simulink model "SWC_TPMS_APS_type"  (R2021b)
settings: Solver=FixedStepDiscrete  StartTime=0.0  StopTime=10.0  FixedStep=0.001  RelTol=1e-3
undefined symbols (not defined in the file or in its folder): f32_ApsOutVehSpdSig, R_HALIN_TPMS_APS_CSOP_PAS_Handler, R_HALIN_TPMS_APS_CSOP_TPMS_Handler, R_HALOUT_TPMS_APS_CSOP_ApsOutput, u8_ApsOutGearPosnSig, u8_ApsOutSendChrgPlugSta, u8_ApsOutSetFrSensorOnCmd, u8_ApsOutSetFrSensorSwTOCmd, u8_ApsOutSetVehSpdTOCmd
(part 1 of 2)
settings Model: DataDictionary=APPTypes.sldd  Creator=FVT23010  LastModifiedBy=FVT23010
settings DataIOCC: SaveFormat=StructureWithTime
settings OptimizationCC: DefaultParameterBehavior=Inlined  EnhancedBackFolding=on  PassReuseOutputArgsAs=Individual arguments  ZeroExternalMemoryAtStartup=off  ZeroInternalMemoryAtStartup=off  OptimizeBlockOrder=speed  DifferentSizesBufferReuse=on  OptimizationCustomize=off  EfficientTunableParamExpr=on
settings DebuggingCC: ParameterTunabilityLossMsg=error
settings HardwareCC: ProdBitPerPointer=32  ProdBitPerSizeT=32  ProdBitPerPtrDiffT=32  ProdLargestAtomicInteger=Long  ProdLargestAtomicFloat=Double  ProdWordSize=32  ProdLongLongMode=on  ProdHWDeviceType=ARM Compatible->ARM Cortex-M
settings ModelReferenceCC: ModelReferenceNumInstancesAllowed=Single
settings SFSimCC: MATLABDynamicMemAlloc=off
settings RTWCC: Description=AUTOSAR  SystemTargetFile=autosar.tlc  GenCodeOnly=on  TemplateMakefile=ert_default_tmf  PortableWordSizes=on
settings CodeAppCC: ForceParamTrailComments=on  IgnoreCustomStorageClasses=off  OperatorAnnotations=on  SimulinkDataObjDesc=on  SFDataObjDesc=on  InsertBlockDesc=on
settings STFCustomTargetCC: TargetLangStandard=C99 (ISO)  MultiwordLength=256  ParMdlRefBuildCompliant=on  CompOptLevelCompliant=on  IncludeMdlTerminateFcn=off  CombineOutputUpdateFcns=on  SuppressErrorStatus=on  ERTCustomFileBanners=on  SupportNonFinite=off  SupportComplex=off  SupportContinuousTime=off  SupportNonInlinedSFcns=off  RemoveResetFunc=on  MATLABClassNameForMDSCustomization=Simulink.SoftwareTarget.ERTCustomization  AutosarCompliant=on  GRTInterface=off  UseToolchainInfoCompliant=on  LookupTableObjectStructAxisOrder=2,1,3,4,...  LUTObjectStructOrderEvenSpacing=Size,Table,Breakpoints  SystemTargetFile=autosar.tlc
settings ERTTargetCC: TargetLangStandard=C99 (ISO)  ConcurrentExecutionCompliant=off  IncludeMdlTerminateFcn=off  SuppressErrorStatus=on  SupportNonFinite=off  SupportComplex=off  ModelStepFunctionPrototypeControlCompliant=off  CPPClassGenCompliant=off  AutosarCompliant=on  LookupTableObjectStructAxisOrder=2,1,3,4,...  LUTObjectStructOrderEvenSpacing=Size,Table,Breakpoints  GenerateASAP2=on  InlinedParameterPlacement=NonHierarchical  ERTCustomFileTemplate=example_file_process.tlc  ConvertIfToSwitch=off  SuppressUnreachableDefaultCases=off  BooleanTrueId=true_MatlabRTW  BooleanFalseId=false_MatlabRTW

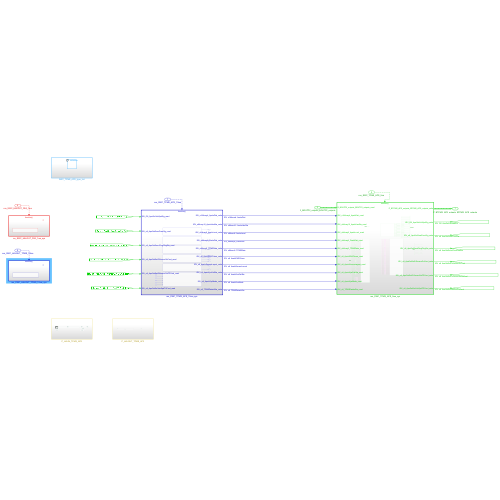
[thumbnail: Simulink's stored preview of the top-level diagram]
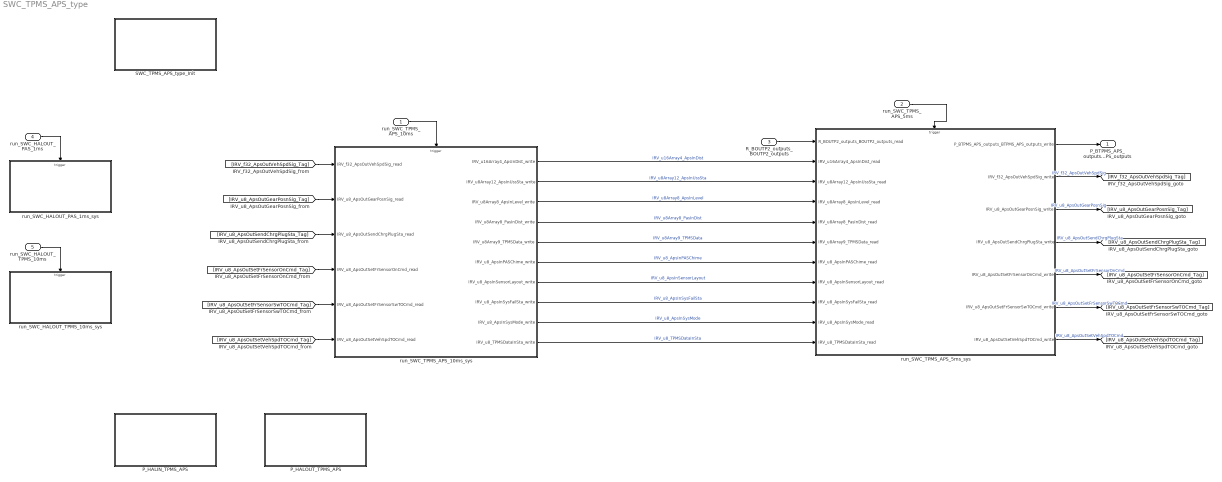
== system SWC_TPMS_APS_type ==
  run_SWC_TPMS_APS_10ms : Inport  SampleTime=0.01  OutputFunctionCall=on
  run_SWC_TPMS_APS_5ms : Inport  Port=2  SampleTime=0.005  OutputFunctionCall=on
  R_BOUTP2_outputs_BOUTP2_outputs : Inport  Port=3  OutDataTypeStr=Bus: BOUTP2_outputs  PortDimensions=1  BusOutputAsStruct=on
  run_SWC_HALOUT_PAS_1ms : Inport  Port=4  SampleTime=0.001  OutputFunctionCall=on
  run_SWC_HALOUT_TPMS_10ms : Inport  Port=5  SampleTime=0.01  OutputFunctionCall=on
  P_HALIN_TPMS_APS : Subsystem
  P_HALOUT_TPMS_APS : Subsystem
  SWC_TPMS_APS_type_Init : Subsystem
  run_SWC_HALOUT_PAS_1ms_sys : Subsystem
  run_SWC_HALOUT_TPMS_10ms_sys : Subsystem
  run_SWC_TPMS_APS_10ms_sys : Subsystem
  run_SWC_TPMS_APS_5ms_sys : Subsystem
  P_BTPMS_APS_outputs_BTPMS_APS_outputs : Outport  OutDataTypeStr=Bus: DT_TPMS_APS_outputs  PortDimensions=1  BusOutputAsStruct=on
  wires:
  R_BOUTP2_outputs_BOUTP2_outputs/1 -> run_SWC_TPMS_APS_5ms_sys/1(R_BOUTP2_outputs_BOUTP2_outputs_read)
  run_SWC_TPMS_APS_5ms_sys/1(P_BTPMS_APS_outputs_BTPMS_APS_outputs_write) -> P_BTPMS_APS_outputs_BTPMS_APS_outputs/1
  run_SWC_TPMS_APS_10ms_sys/1(IRV_u16Array4_ApsInDist_write) -> run_SWC_TPMS_APS_5ms_sys/2(IRV_u16Array4_ApsInDist_read)  "IRV_u16Array4_ApsInDist"
  run_SWC_TPMS_APS_10ms_sys/2(IRV_u8Array12_ApsInUssSta_write) -> run_SWC_TPMS_APS_5ms_sys/3(IRV_u8Array12_ApsInUssSta_read)  "IRV_u8Array12_ApsInUssSta"
  run_SWC_TPMS_APS_10ms_sys/3(IRV_u8Array8_ApsInLevel_write) -> run_SWC_TPMS_APS_5ms_sys/4(IRV_u8Array8_ApsInLevel_read)  "IRV_u8Array8_ApsInLevel"
  run_SWC_TPMS_APS_10ms_sys/4(IRV_u8Array8_PasInDist_write) -> run_SWC_TPMS_APS_5ms_sys/5(IRV_u8Array8_PasInDist_read)  "IRV_u8Array8_PasInDist"
  run_SWC_TPMS_APS_10ms_sys/5(IRV_u8Array9_TPMSData_write) -> run_SWC_TPMS_APS_5ms_sys/6(IRV_u8Array9_TPMSData_read)  "IRV_u8Array9_TPMSData"
  run_SWC_TPMS_APS_10ms_sys/6(IRV_u8_ApsInPASChime_write) -> run_SWC_TPMS_APS_5ms_sys/7(IRV_u8_ApsInPASChime_read)  "IRV_u8_ApsInPASChime"
  run_SWC_TPMS_APS_10ms_sys/7(IRV_u8_ApsInSensorLayout_write) -> run_SWC_TPMS_APS_5ms_sys/8(IRV_u8_ApsInSensorLayout_read)  "IRV_u8_ApsInSensorLayout"
  run_SWC_TPMS_APS_10ms_sys/8(IRV_u8_ApsInSysFailSta_write) -> run_SWC_TPMS_APS_5ms_sys/9(IRV_u8_ApsInSysFailSta_read)  "IRV_u8_ApsInSysFailSta"
  run_SWC_TPMS_APS_10ms_sys/9(IRV_u8_ApsInSysMode_write) -> run_SWC_TPMS_APS_5ms_sys/10(IRV_u8_ApsInSysMode_read)  "IRV_u8_ApsInSysMode"
  run_SWC_TPMS_APS_10ms_sys/10(IRV_u8_TPMSDataInSta_write) -> run_SWC_TPMS_APS_5ms_sys/11(IRV_u8_TPMSDataInSta_read)  "IRV_u8_TPMSDataInSta"
  run_SWC_TPMS_APS_5ms_sys/7(IRV_u8_ApsOutSetVehSpdTOCmd_write) -> [IRV_u8_ApsOutSetVehSpdTOCmd_Tag]  "IRV_u8_ApsOutSetVehSpdTOCmd"
  [IRV_u8_ApsOutSetVehSpdTOCmd_Tag] -> run_SWC_TPMS_APS_10ms_sys/6(IRV_u8_ApsOutSetVehSpdTOCmd_read)
  run_SWC_TPMS_APS_5ms_sys/6(IRV_u8_ApsOutSetFrSensorSwTOCmd_write) -> [IRV_u8_ApsOutSetFrSensorSwTOCmd_Tag]  "IRV_u8_ApsOutSetFrSensorSwTOCmd"
  [IRV_u8_ApsOutSetFrSensorSwTOCmd_Tag] -> run_SWC_TPMS_APS_10ms_sys/5(IRV_u8_ApsOutSetFrSensorSwTOCmd_read)
  run_SWC_TPMS_APS_5ms_sys/5(IRV_u8_ApsOutSetFrSensorOnCmd_write) -> [IRV_u8_ApsOutSetFrSensorOnCmd_Tag]  "IRV_u8_ApsOutSetFrSensorOnCmd"
  [IRV_u8_ApsOutSetFrSensorOnCmd_Tag] -> run_SWC_TPMS_APS_10ms_sys/4(IRV_u8_ApsOutSetFrSensorOnCmd_read)
  run_SWC_TPMS_APS_5ms_sys/4(IRV_u8_ApsOutSendChrgPlugSta_write) -> [IRV_u8_ApsOutSendChrgPlugSta_Tag]  "IRV_u8_ApsOutSendChrgPlugSta"
  [IRV_u8_ApsOutSendChrgPlugSta_Tag] -> run_SWC_TPMS_APS_10ms_sys/3(IRV_u8_ApsOutSendChrgPlugSta_read)
  run_SWC_TPMS_APS_5ms_sys/3(IRV_u8_ApsOutGearPosnSig_write) -> [IRV_u8_ApsOutGearPosnSig_Tag]  "IRV_u8_ApsOutGearPosnSig"
  [IRV_u8_ApsOutGearPosnSig_Tag] -> run_SWC_TPMS_APS_10ms_sys/2(IRV_u8_ApsOutGearPosnSig_read)
  run_SWC_TPMS_APS_5ms_sys/2(IRV_f32_ApsOutVehSpdSig_write) -> [IRV_f32_ApsOutVehSpdSig_Tag]  "IRV_f32_ApsOutVehSpdSig"
  [IRV_f32_ApsOutVehSpdSig_Tag] -> run_SWC_TPMS_APS_10ms_sys/1(IRV_f32_ApsOutVehSpdSig_read)
  run_SWC_TPMS_APS_10ms/1 -> run_SWC_TPMS_APS_10ms_sys/Trigger
  run_SWC_TPMS_APS_5ms/1 -> run_SWC_TPMS_APS_5ms_sys/Trigger
  run_SWC_HALOUT_PAS_1ms/1 -> run_SWC_HALOUT_PAS_1ms_sys/Trigger
  run_SWC_HALOUT_TPMS_10ms/1 -> run_SWC_HALOUT_TPMS_10ms_sys/Trigger

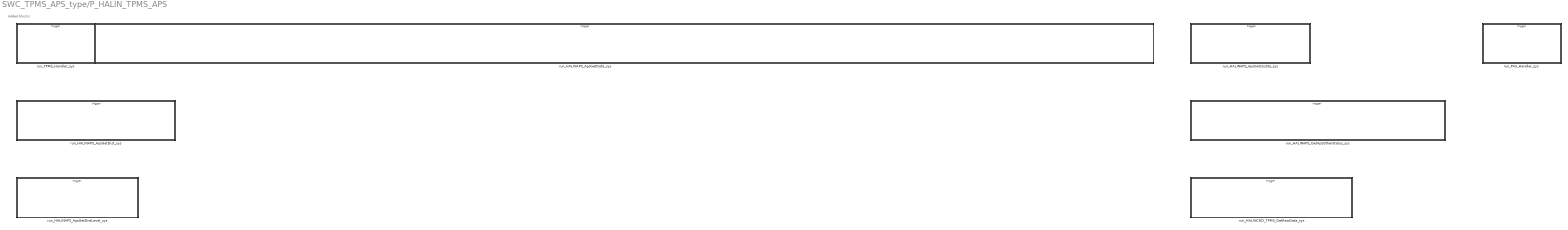
== system SWC_TPMS_APS_type/P_HALIN_TPMS_APS ==
  note: Added blocks
  run_HALINAPS_ApsGetData_sys : Subsystem
  run_HALINAPS_ApsGetDistLevel_sys : Subsystem
  run_HALINAPS_ApsGetDist_sys : Subsystem
  run_HALINAPS_ApsGetUssSta_sys : Subsystem
  run_HALINAPS_GetApsOtherStatus_sys : Subsystem
  run_HALINCDD_TPMS_GetRawData_sys : Subsystem
  run_PAS_Handler_sys : Subsystem
  run_TPMS_Handler_sys : Subsystem

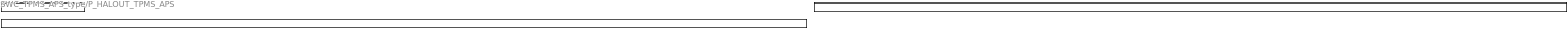
== system SWC_TPMS_APS_type/P_HALOUT_TPMS_APS ==
  run_HALOUTAPS_ApsOutput_sys : Subsystem
  run_HALOUTAPS_ApsSetData_sys : Subsystem
  run_HALOUTAPS_ApsSetTimeout_sys : Subsystem

== system SWC_TPMS_APS_type/SWC_TPMS_APS_type_Init ==
  Event Listener : EventListener  EventName=reset

== system SWC_TPMS_APS_type/run_SWC_HALOUT_PAS_1ms_sys ==
  function : TriggerPort  TriggerType=function-call  VariantControl=(inherit)  SampleTimeType=periodic  SampleTime=-1
  R_HALIN_TPMS_APS_CSOP_PAS_Handler : FunctionCaller  FunctionPrototype=R_HALIN_TPMS_APS_CSOP_PAS_Handler()

== system SWC_TPMS_APS_type/run_SWC_HALOUT_TPMS_10ms_sys ==
  function : TriggerPort  TriggerType=function-call  VariantControl=(inherit)  SampleTimeType=periodic  SampleTime=-1
  R_HALIN_TPMS_APS_CSOP_TPMS_Handler : FunctionCaller  FunctionPrototype=R_HALIN_TPMS_APS_CSOP_TPMS_Handler()

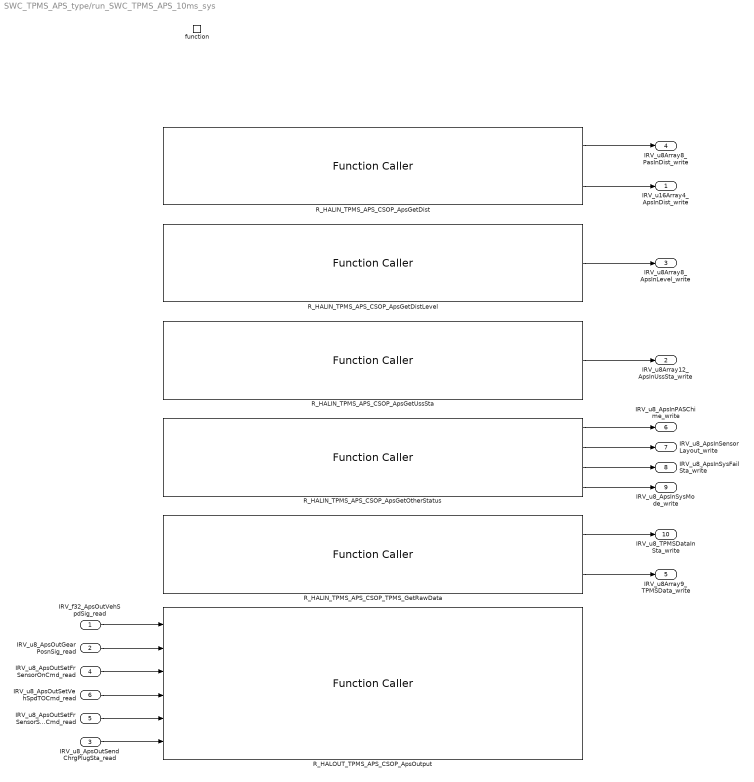
== system SWC_TPMS_APS_type/run_SWC_TPMS_APS_10ms_sys ==
  IRV_f32_ApsOutVehSpdSig_read : Inport
  IRV_u8_ApsOutGearPosnSig_read : Inport  Port=2
  IRV_u8_ApsOutSendChrgPlugSta_read : Inport  Port=3
  IRV_u8_ApsOutSetFrSensorOnCmd_read : Inport  Port=4
  IRV_u8_ApsOutSetFrSensorSwTOCmd_read : Inport  Port=5
  IRV_u8_ApsOutSetVehSpdTOCmd_read : Inport  Port=6
  function : TriggerPort  TriggerType=function-call  VariantControl=(inherit)  SampleTimeType=periodic  SampleTime=-1
  R_HALIN_TPMS_APS_CSOP_ApsGetDist : FunctionCaller  FunctionPrototype=[u8Array8_PasInDist,u16Array4_ApsInDist] = R_HALIN_TPMS_APS_CSOP_ApsGetDist()  OutputArgumentSpecifications=uint8([1;1;1;1;1;1;1;1]), uint16([1;1;1;1])
  R_HALIN_TPMS_APS_CSOP_ApsGetDistLevel : FunctionCaller  FunctionPrototype=u8Array8_ApsInLevel = R_HALIN_TPMS_APS_CSOP_ApsGetDistLevel()  OutputArgumentSpecifications=uint8([1;1;1;1;1;1;1;1])
  R_HALIN_TPMS_APS_CSOP_ApsGetOtherStatus : FunctionCaller  FunctionPrototype=[u8_ApsInPASChime,u8_ApsInSensorLayout,u8_ApsInSysFailSta,u8_ApsInSysMode] = R_HALIN_TPMS_APS_CSOP_ApsGetOtherStatus()  OutputArgumentSpecifications=uint8(1), uint8(1), uint8(1), uint8(1)
  R_HALIN_TPMS_APS_CSOP_ApsGetUssSta : FunctionCaller  FunctionPrototype=u8Array12_ApsInUssSta = R_HALIN_TPMS_APS_CSOP_ApsGetUssSta()  OutputArgumentSpecifications=uint8([1;1;1;1;1;1;1;1;1;1;1;1])
  R_HALIN_TPMS_APS_CSOP_TPMS_GetRawData : FunctionCaller  FunctionPrototype=[u8_TPMSDataInSta,u8Array9_TPMSData] = R_HALIN_TPMS_APS_CSOP_TPMS_GetRawData()  OutputArgumentSpecifications=uint8(1), uint8([1;1;1;1;1;1;1;1;1])
  R_HALOUT_TPMS_APS_CSOP_ApsOutput : FunctionCaller  FunctionPrototype=R_HALOUT_TPMS_APS_CSOP_ApsOutput(f32_ApsOutVehSpdSig,u8_ApsOutGearPosnSig,u8_ApsOutSetFrSensorOnCmd,u8_ApsOutSetVehSpdTOCmd,u8_ApsOutSetFrSensorSwTOCmd,u8_ApsOutSendChrgPlugSta)  InputArgumentSpecifications=single(1), uint8(1), uint8(1), uint8(1), uint8(1), uint8(1)
  IRV_u16Array4_ApsInDist_write : Outport  OutDataTypeStr=uint16  PortDimensions=4
  IRV_u8Array12_ApsInUssSta_write : Outport  Port=2  OutDataTypeStr=uint8  PortDimensions=12
  IRV_u8Array8_ApsInLevel_write : Outport  Port=3  OutDataTypeStr=uint8  PortDimensions=8
  IRV_u8Array8_PasInDist_write : Outport  Port=4  OutDataTypeStr=uint8  PortDimensions=8
  IRV_u8Array9_TPMSData_write : Outport  Port=5  OutDataTypeStr=uint8  PortDimensions=9
  IRV_u8_ApsInPASChime_write : Outport  Port=6  OutDataTypeStr=uint8  PortDimensions=1
  IRV_u8_ApsInSensorLayout_write : Outport  Port=7  OutDataTypeStr=uint8  PortDimensions=1
  IRV_u8_ApsInSysFailSta_write : Outport  Port=8  OutDataTypeStr=uint8  PortDimensions=1
  IRV_u8_ApsInSysMode_write : Outport  Port=9  OutDataTypeStr=uint8  PortDimensions=1
  IRV_u8_TPMSDataInSta_write : Outport  Port=10  OutDataTypeStr=uint8  PortDimensions=1
  wires:
  R_HALIN_TPMS_APS_CSOP_ApsGetDist/1 -> IRV_u8Array8_PasInDist_write/1
  R_HALIN_TPMS_APS_CSOP_ApsGetDist/2 -> IRV_u16Array4_ApsInDist_write/1
  R_HALIN_TPMS_APS_CSOP_ApsGetDistLevel/1 -> IRV_u8Array8_ApsInLevel_write/1
  R_HALIN_TPMS_APS_CSOP_ApsGetUssSta/1 -> IRV_u8Array12_ApsInUssSta_write/1
  R_HALIN_TPMS_APS_CSOP_ApsGetOtherStatus/1 -> IRV_u8_ApsInPASChime_write/1
  R_HALIN_TPMS_APS_CSOP_ApsGetOtherStatus/2 -> IRV_u8_ApsInSensorLayout_write/1
  R_HALIN_TPMS_APS_CSOP_ApsGetOtherStatus/3 -> IRV_u8_ApsInSysFailSta_write/1
  R_HALIN_TPMS_APS_CSOP_ApsGetOtherStatus/4 -> IRV_u8_ApsInSysMode_write/1
  R_HALIN_TPMS_APS_CSOP_TPMS_GetRawData/1 -> IRV_u8_TPMSDataInSta_write/1
  R_HALIN_TPMS_APS_CSOP_TPMS_GetRawData/2 -> IRV_u8Array9_TPMSData_write/1
  IRV_f32_ApsOutVehSpdSig_read/1 -> R_HALOUT_TPMS_APS_CSOP_ApsOutput/1
  IRV_u8_ApsOutGearPosnSig_read/1 -> R_HALOUT_TPMS_APS_CSOP_ApsOutput/2
  IRV_u8_ApsOutSetFrSensorOnCmd_read/1 -> R_HALOUT_TPMS_APS_CSOP_ApsOutput/3
  IRV_u8_ApsOutSetVehSpdTOCmd_read/1 -> R_HALOUT_TPMS_APS_CSOP_ApsOutput/4
  IRV_u8_ApsOutSetFrSensorSwTOCmd_read/1 -> R_HALOUT_TPMS_APS_CSOP_ApsOutput/5
  IRV_u8_ApsOutSendChrgPlugSta_read/1 -> R_HALOUT_TPMS_APS_CSOP_ApsOutput/6

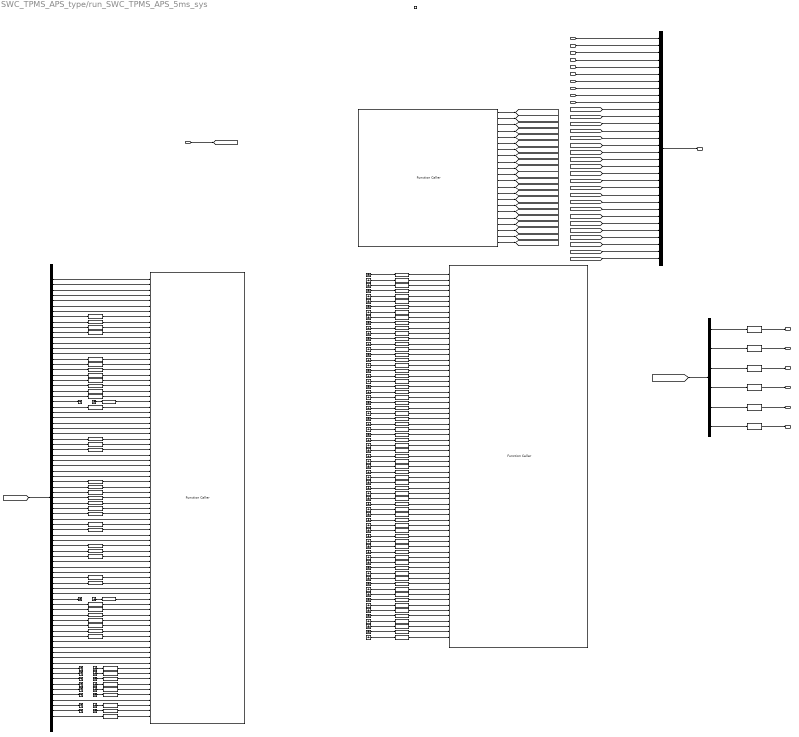
== system SWC_TPMS_APS_type/run_SWC_TPMS_APS_5ms_sys ==
  R_BOUTP2_outputs_BOUTP2_outputs_read : Inport
  IRV_u16Array4_ApsInDist_read : Inport  Port=2
  IRV_u8Array12_ApsInUssSta_read : Inport  Port=3
  IRV_u8Array8_ApsInLevel_read : Inport  Port=4
  IRV_u8Array8_PasInDist_read : Inport  Port=5
  IRV_u8Array9_TPMSData_read : Inport  Port=6
  IRV_u8_ApsInPASChime_read : Inport  Port=7
  IRV_u8_ApsInSensorLayout_read : Inport  Port=8
  IRV_u8_ApsInSysFailSta_read : Inport  Port=9
  IRV_u8_ApsInSysMode_read : Inport  Port=10
  IRV_u8_TPMSDataInSta_read : Inport  Port=11
  function : TriggerPort  TriggerType=function-call  VariantControl=(inherit)  SampleTimeType=periodic  SampleTime=-1
  Bus Creator : BusCreator  Inputs=32  OutDataTypeStr=Bus: DT_TPMS_APS_outputs  NonVirtualBus=on
  Bus Selector : BusSelector  OutputSignals=VOUTP_VehSpeed_kph,VOUTP_ShiftGearPosn_enum,VOUTP_FSOffSw_enum,VOUTP_VehSpeedTimeOut_flg,VOUTP_FSOffSwTimeOut_flg,VOUTP_ChrgPlugSta_enum
  Bus Selector3 : BusSelector  OutputSignals=VOUTP_PowerSta_enum,VOUTP_BrkPedalPos_pct,VOUTP_ActAPSPosn_pct,VOUTP_LFRawWhlSpeed_kph,VOUTP_RFRawWhlSpeed_kph,VOUTP_LRRawWhlSpeed_kph,VOUTP_RRRawWhlSpeed_kph,VOUTP_LFRawWhlSpeedV_flg,VOUTP_RFRawWhlSpeedV_flg,VOUTP_LRRawWhlSpeedV_flg,VOUTP_RRRawWhlSpeedV_flg,VOUTP_LFWhlRotDir_enum,VOUTP_RFWhlRotDir_enum,VOUTP_LRWhlRotDir_enum,VOUTP_RRWhlRotDir_enum,VOUTP_LFPulseCountV_flg,VOUTP_RFPulseCountV_flg,VOUTP_LRPulseCountV_flg,VOUTP_RRPulseCountV_flg,VOUTP_LFPulseCount_enum,VOUTP_RFPulseCount_enum,VOUTP_LRPulseCount_enum,VOUTP_RRPulseCount_enum,VOUTP_VehSpeed_kph,VOUTP_APSCtrlAvail_flg,VOUTP_ShifterHandleCmd_enum,VOUTP_DriIntend_enum,VOUTP_EPSAOIControl_enum,VOUTP_SASAngle_Deg,VOUTP_SASSpeed_degps,VOUTP_SASSpeedValid_flg,VOUTP_SASCAL_flg,VOUTP_SASV_flg,VOUTP_GRADE_Deg,VOUTP_YawRate_degps,VOUTP_LatAccel_Gps,VOUTP_LongAccel_Gps,VOUTP_MCPressure_bar,VOUTP_YawRateV_flg,VOUTP_LatAccelV_flg,VOUTP_LongAccelV_flg,VOUTP_MCPressureV_bar,VOUTP_BrkSwSta_flg,VOUTP_BrkSwV_flg,VOUTP_ESCStandstill_flg,VOUTP_ESCAPSSta_enum,VOUTP_EPBExtReleaseAvail_flg,VOUTP_EPBExtApplyAvail_flg,VOUTP_EPBErrSta_enum,VOUTP_EPBSta_enum,VOUTP_AllDoorSW_flg,VOUTP_HoodSW_flg,VOUTP_TailgateSW_flg,VOUTP_AVMparkingcancel_enum,VOUTP_AVMparkingexcute_enum,VOUTP_AVMParkingmode_enum,VOUTP_AVMErrSTA_flg,VOUTP_IVIStatus_flg,VOUTP_CAASSw_enum,VOUTP_IVIScreen_enum,VOUTP_VehSpeedTimeOut_flg,VOUTP_ABSActive_flg,VOUTP_TCSActive_flg,VOUTP_DriverSeatBeltCmd_flg,VOUTP_DrDoorSW_flg,VOUTP_PsDoorSW_flg,VOUTP_RLDoorSW_flg,VOUTP_RRDoorSW_flg,VOUTP_RFPressIndi_enum,VOUTP_LFPressIndi_enum,VOUTP_RRPressIndi_enum,VOUTP_LRPressIndi_enum,VOUTP_sigAmbAirT_C,VOUTP_FSOffSw_enum,VOUTP_FSOffSwTimeOut_flg,VOUTP_VehSpeed_kph,VOUTP_VehSpeed_kph,VOUTP_VehSpeed_kph,VOUTP_VehSpeed_kph,VOUTP_DrSeatSta_enum,VOUTP_VehSpeed_kph,VOUTP_VehSpeed_kph,VOUTP_IVIUserTakeOverAPSSta_flg
  Data Type Conversion : DataTypeConversion  OutDataTypeStr=single
  Data Type Conversion{1..5,7..13,17..19,21..106,109..124} (117 alike) : DataTypeConversion  OutDataTypeStr=uint8
  Data Type Conversion{14..16,20} (4 alike) : DataTypeConversion  OutDataTypeStr=int16
  Data Type Conversion6 : DataTypeConversion  OutDataTypeStr=single
  Ground{,1..32} (33 alike) : Ground
  Ground_{1..46} (46 alike) : Ground
  R_HALIN_TPMS_APS_CSOP_ApsGetData : FunctionCaller  FunctionPrototype=[u8_GetAPS_Progress_PCT,u8_GetAPS_RQ_Display,u8_GetAPS_SW_Ver,u8_GetAPS_HW_Ver,u8_GetAPS_ExitCondition,f32_GetAPS_Angle_Target,u8_GetAPS_Sta_System,u8_GetAPS_V_Rq_EPAS_Ctrl,u8_GetAPS_Rq_EPAS_Ctrl,u8_GetAPS_Req,f32_GetAPS_DecReq,u8_GetAPS_DecReq_A,f32_GetAPS_SpeedCmd,u8_GetAPS_ShftPosnReq,u8_GetAPS_VMC_Req_A,u8_GetCAAS_Sta,u8_GetCAAS_VMC_Req_A,u8_GetAPS_PwrReq_cmd,u8_GetRAPS_BCM_LockReq_Cmd,u8_GetRAPS_BCM_Lamp_Cmd,u8_GetRAPS_ErrWarn_Sta,u8_GetRAPS_ErrLv1_flg] = R_HALIN_TPMS_APS_CSOP_ApsGetData()  OutputArgumentSpecifications=uint8(1), uint8(1), uint8(1), uint8(1), uint8(1), single(1), uint8(1), uint8(1), uint8(1), uint8(1), single(1), uint8(1), single(1), uint8(1), uint8(1), uint8(1), uint8(1), uint8(1), uint8(1), uint8(1), uint8(1), uint8(1)
  R_HALOUT_TPMS_APS_CSOP_ApsSetData : FunctionCaller  FunctionPrototype=R_HALOUT_TPMS_APS_CSOP_ApsSetData(u8_SetPwrSta,f32_SetBrkPedalPos,f32_SetActAPSPosn,f32_SetLF_RawWhlSpeed,f32_SetRF_RawWhlSpeed,f32_SetLR_RawWhlSpeed,f32_SetRR_RawWhlSpeed,u8_SetLF_RawWhlSpeed_V,u8_SetRF_RawWhlSpeed_V,u8_SetLR_RawWhlSpeed_V,u8_SetRR_RawWhlSpeed_V,u8_SetLF_WhlRotDir,u8_SetRF_WhlRotDir,u8_SetLR_WhlRotDir,u8_SetRR_WhlRotDir,u8_SetLF_PulseCount_V,u8_SetRF_PulseCount_V,u8_SetLR_PulseCount_V,u8_SetRR_PulseCount_V,s16_SetLF_PulseCount,s16_SetRF_PulseCount,s16_SetLR_PulseCount,s16_SetRR_PulseCount,u8_SetAPS_Active,u8_SetAPS_CtrlAvail,u8_SetShifter_Handle_Cmd,u8_SetDriIntend,u8_SetEPS_AOI_Control,f32_SetSAS_Angle,f32_SetSAS_Speed,u8_SetSAS_Speed_Valid,u8_SetSAS_CAL,u8_SetSAS_OK,f32_SetGRADE,f32_SetYawRate,f32_SetLatAccel,f32_SetLongAccel,f32_SetMCPressure,u8_SetYawRate_V,u8_SetLatAccel_V,u8_SetLongAccel_V,u8_SetMCPressure_V,u8_SetBrkSw_Sta,u8_SetBrkSw_V,u8_SetESC_Standstill,u8_SetESC_APS_Sta,u8_SetEPBExtReleaseAvail,u8_SetEPBExtApplyAvail,u8_SetEPBErrSta,u8_SetEPBSta,u8_SetAllDoorSW,u8_SetHoodSW,u8_SetTailgate_SW,u8_SetAVM_parking_cancel,u8_SetAVM_parking_excute,u8_SetAVM_Parking_mode,u8_SetAVM_Err_STA,u8_SetIVI_Status,u8_SetCAAS_Sw,u8_SetIVI_Screen,u8_SetCAAS_CtrlAvail,u8_SetABS_Active,u8_SetTCS_Active,u8_SetDriverSeatBeltCmd,u8_SetDrDoorSW,u8_SetPsDoorSW,u8_SetRLDoorSW,u8_SetRRDoorSW,u8_SetRFPressIndi,u8_SetLFPressIndi,u8_SetRRPressIndi,u8_SetLRPressIndi,f32_SetsigAmbAirT,f32_SetVehActSpd,u8_SetCAAS_Active,u8_SetAPS_PwrReqAvail_sta,u8_SetDKC_PDkeyAreaRAPS_Sta,u8_SetDKC_ParkingMode_Cmd,u8_SetP_UID_LowPower,u8_SetDr_SeatSta,u8_SetVCU_RAPSErrLv2_flg,u8_SetVCU_RAPSErrLv3_flg,u8_SetIVI_UserTakeOver_APS_Sta)  InputArgumentSpecifications=uint8(1), single(1), single(1), single(1), single(1), single(1), single(1), uint8(1), uint8(1), uint8(1), uint8(1), uint8(1), uint8(1), uint8(1), uint8(1), uint8(1), uint8(1), uint8(1), uint8(1), int16(1), int16(1), int16(1), int16(1), uint8(1), uint8(1), uint8(1), uint8(1), uint8(1), single(1), single(1), uint8(1), uint8(1), uint8(1), single(1), single(1), single(1), single(1), single(1), uint8(1), uint8(1), uint8(1), uint8(1), uint8(1), uint8(1), uint8(1), uint8(1), uint8(1), uint8(1), uint8(1), uint8(1), uint8(1), uint8(1), uint8(1), uint8(1), uint8(1), uint8(1), uint8(1), uint8(1), uint8(1), uint8(1), uint8(1), uint8(1), uint8(1), uint8(1), uint8(1), uint8(1), uint8(1), uint8(1), uint8(1), uint8(1), uint8(1), uint8(1), single(1), single(1), uint8(1), uint8(1), uint8(1), uint8(1), uint8(1), uint8(1), uint8(1), uint8(1), uint8(1)
  R_HALOUT_TPMS_APS_CSOP_ApsSetTimeout : FunctionCaller  FunctionPrototype=R_HALOUT_TPMS_APS_CSOP_ApsSetTimeout(u8_SetBrkPedalPosTO,u8_SetLF_RawWhlSpeedTO,u8_SetRF_RawWhlSpeedTO,u8_SetLR_RawWhlSpeedTO,u8_SetRR_RawWhlSpeedTO,u8_SetLF_RawWhlSpeed_VTO,u8_SetRF_RawWhlSpeed_VTO,u8_SetLR_RawWhlSpeed_VTO,u8_SetRR_RawWhlSpeed_VTO,u8_SetLF_WhlRotDirTO,u8_SetRF_WhlRotDirTO,u8_SetLR_WhlRotDirTO,u8_SetRR_WhlRotDirTO,u8_SetLF_PulseCount_VTO,u8_SetRF_PulseCount_VTO,u8_SetLR_PulseCount_VTO,u8_SetRR_PulseCount_VTO,u8_SetLF_PulseCountTO,u8_SetRF_PulseCountTO,u8_SetLR_PulseCountTO,u8_SetRR_PulseCountTO,u8_SetShifter_Handle_CmdTO,u8_SetDriIntendTO,u8_SetEPS_AOI_ControlTO,u8_SetSAS_AngleTO,u8_SetSAS_SpeedTO,u8_SetSAS_Speed_ValidTO,u8_SetSAS_CALTO,u8_SetSAS_OKTO,u8_SetGRADETO,u8_SetYawRateTO,u8_SetLatAccelTO,u8_SetLongAccelTO,u8_SetMCPressureTO,u8_SetYawRate_VTO,u8_SetLatAccel_VTO,u8_SetLongAccel_VTO,u8_SetMCPressure_VTO,u8_SetBrkSw_StaTO,u8_SetBrkSw_VTO,u8_SetESC_StandstillTO,u8_SetESC_APS_StaTO,u8_SetEPBExtReleaseAvailTO,u8_SetEPBExtApplyAvailTO,u8_SetEPBErrStaTO,u8_SetEPBStaTO,u8_SetAVM_parking_cancelTO,u8_SetAVM_parking_excuteTO,u8_SetAVM_Parking_modeTO,u8_SetAVM_Err_STATO,u8_SetIVI_StatusTO,u8_SetCAAS_SwTO,u8_SetIVI_ScreenTO,u8_SetABS_ActiveTO,u8_SetTCS_ActiveTO,u8_SetDriverSeatBeltCmdTO,u8_SetRFPressIndiTO,u8_SetLFPressIndiTO,u8_SetRRPressIndiTO,u8_SetLRPressIndiTO,u8_SetsigAmbAirTTO,u8_SetAPS_PwrReqAvail_staTO,u8_SetDKC_PDkeyAreaRAPS_StaTO,u8_SetDKC_ParkingMode_CmdTO,u8_SetP_UID_LowPowerTO,u8_SetDr_SeatStaTO,u8_SetVCU_RAPSErrLv2_flgTO,u8_SetVCU_RAPSErrLv3_flgTO,u8_SetIVI_UserTakeOver_APS_StaTO)  InputArgumentSpecifications=uint8(1), uint8(1), uint8(1), uint8(1), uint8(1), uint8(1), uint8(1), uint8(1), uint8(1), uint8(1), uint8(1), uint8(1), uint8(1), uint8(1), uint8(1), uint8(1), uint8(1), uint8(1), uint8(1), uint8(1), uint8(1), uint8(1), uint8(1), uint8(1), uint8(1), uint8(1), uint8(1), uint8(1), uint8(1), uint8(1), uint8(1), uint8(1), uint8(1), uint8(1), uint8(1), uint8(1), uint8(1), uint8(1), uint8(1), uint8(1), uint8(1), uint8(1), uint8(1), uint8(1), uint8(1), uint8(1), uint8(1), uint8(1), uint8(1), uint8(1), uint8(1), uint8(1), uint8(1), uint8(1), uint8(1), uint8(1), uint8(1), uint8(1), uint8(1), uint8(1), uint8(1), uint8(1), uint8(1), uint8(1), uint8(1), uint8(1), uint8(1), uint8(1), uint8(1)
  Terminator{,6..8,10..15} (10 alike) : Terminator
  P_BTPMS_APS_outputs_BTPMS_APS_outputs_write : Outport
  IRV_f32_ApsOutVehSpdSig_write : Outport  Port=2  OutDataTypeStr=single  PortDimensions=1
  IRV_u8_ApsOutGearPosnSig_write : Outport  Port=3  OutDataTypeStr=uint8  PortDimensions=1
  IRV_u8_ApsOutSendChrgPlugSta_write : Outport  Port=4  OutDataTypeStr=uint8  PortDimensions=1
  IRV_u8_ApsOutSetFrSensorOnCmd_write : Outport  Port=5  OutDataTypeStr=uint8  PortDimensions=1
  IRV_u8_ApsOutSetFrSensorSwTOCmd_write : Outport  Port=6  OutDataTypeStr=uint8  PortDimensions=1
  IRV_u8_ApsOutSetVehSpdTOCmd_write : Outport  Port=7  OutDataTypeStr=uint8  PortDimensions=1
  wires:
  R_HALIN_TPMS_APS_CSOP_ApsGetData/2 -> [u8_GetAPS_RQ_Display]
  R_HALIN_TPMS_APS_CSOP_ApsGetData/15 -> [u8_GetAPS_VMC_Req_A]
  R_HALIN_TPMS_APS_CSOP_ApsGetData/19 -> [u8_GetRAPS_BCM_LockReq_Cmd]
  R_HALIN_TPMS_APS_CSOP_ApsGetData/4 -> [u8_GetAPS_HW_Ver]
  R_HALIN_TPMS_APS_CSOP_ApsGetData/3 -> [u8_GetAPS_SW_Ver]
  R_HALIN_TPMS_APS_CSOP_ApsGetData/11 -> [f32_GetAPS_DecReq]
  R_HALIN_TPMS_APS_CSOP_ApsGetData/21 -> [u8_GetRAPS_ErrWarn_Sta]
  R_HALIN_TPMS_APS_CSOP_ApsGetData/16 -> [u8_GetCAAS_Sta]
  R_HALIN_TPMS_APS_CSOP_ApsGetData/14 -> [u8_GetAPS_ShftPosnReq]
  R_HALIN_TPMS_APS_CSOP_ApsGetData/13 -> [f32_GetAPS_SpeedCmd]
  R_HALIN_TPMS_APS_CSOP_ApsGetData/6 -> [f32_GetAPS_Angle_Target]
  R_HALIN_TPMS_APS_CSOP_ApsGetData/20 -> [u8_GetRAPS_BCM_Lamp_Cmd]
  R_HALIN_TPMS_APS_CSOP_ApsGetData/7 -> [u8_GetAPS_Sta_System]
  R_HALIN_TPMS_APS_CSOP_ApsGetData/1 -> [u8_GetAPS_Progress_PCT]
  R_HALIN_TPMS_APS_CSOP_ApsGetData/10 -> [u8_GetAPS_Req]
  R_HALIN_TPMS_APS_CSOP_ApsGetData/18 -> [u8_GetAPS_PwrReq_cmd]
  R_HALIN_TPMS_APS_CSOP_ApsGetData/22 -> [u8_GetRAPS_ErrLv1_flg]
  R_HALIN_TPMS_APS_CSOP_ApsGetData/8 -> [u8_GetAPS_V_Rq_EPAS_Ctrl]
  R_HALIN_TPMS_APS_CSOP_ApsGetData/5 -> [u8_GetAPS_ExitCondition]
  R_HALIN_TPMS_APS_CSOP_ApsGetData/12 -> [u8_GetAPS_DecReq_A]
  R_HALIN_TPMS_APS_CSOP_ApsGetData/17 -> [u8_GetCAAS_VMC_Req_A]
  R_HALIN_TPMS_APS_CSOP_ApsGetData/9 -> [u8_GetAPS_Rq_EPAS_Ctrl]
  [u8_GetAPS_Progress_PCT] -> Bus Creator/11
  [u8_GetAPS_PwrReq_cmd] -> Bus Creator/28
  [f32_GetAPS_Angle_Target] -> Bus Creator/16
  [u8_GetCAAS_VMC_Req_A] -> Bus Creator/27
  [u8_GetAPS_Sta_System] -> Bus Creator/17
  Bus Creator/1 -> P_BTPMS_APS_outputs_BTPMS_APS_outputs_write/1
  [u8_GetRAPS_BCM_Lamp_Cmd] -> Bus Creator/30
  [u8_GetAPS_V_Rq_EPAS_Ctrl] -> Bus Creator/18
  [u8_GetAPS_Req] -> Bus Creator/20
  [u8_GetRAPS_BCM_LockReq_Cmd] -> Bus Creator/29
  [u8_GetRAPS_ErrWarn_Sta] -> Bus Creator/31
  [u8_GetRAPS_ErrLv1_flg] -> Bus Creator/32
  [u8_GetAPS_DecReq_A] -> Bus Creator/22
  [u8_GetAPS_SW_Ver] -> Bus Creator/13
  [f32_GetAPS_SpeedCmd] -> Bus Creator/23
  [u8_GetCAAS_Sta] -> Bus Creator/26
  [u8_GetAPS_VMC_Req_A] -> Bus Creator/25
  [u8_GetAPS_ExitCondition] -> Bus Creator/15
  [u8_GetAPS_ShftPosnReq] -> Bus Creator/24
  [u8_GetAPS_Rq_EPAS_Ctrl] -> Bus Creator/19
  [u8_GetAPS_RQ_Display] -> Bus Creator/12
  [f32_GetAPS_DecReq] -> Bus Creator/21
  [u8_GetAPS_HW_Ver] -> Bus Creator/14
  IRV_u8Array9_TPMSData_read/1 -> Bus Creator/5
  IRV_u8_ApsInPASChime_read/1 -> Bus Creator/6
  IRV_u8_ApsInSensorLayout_read/1 -> Bus Creator/7
  IRV_u8Array8_ApsInLevel_read/1 -> Bus Creator/3
  IRV_u8Array8_PasInDist_read/1 -> Bus Creator/4
  IRV_u8_ApsInSysFailSta_read/1 -> Bus Creator/8
  IRV_u8_ApsInSysMode_read/1 -> Bus Creator/9
  IRV_u16Array4_ApsInDist_read/1 -> Bus Creator/1
  IRV_u8Array12_ApsInUssSta_read/1 -> Bus Creator/2
  IRV_u8_TPMSDataInSta_read/1 -> Bus Creator/10
  Bus Selector3/8 -> Data Type Conversion7/1  "<VOUTP_LFRawWhlSpeedV_flg>"
  Data Type Conversion99/1 -> R_HALOUT_TPMS_APS_CSOP_ApsSetData/67
  Data Type Conversion102/1 -> R_HALOUT_TPMS_APS_CSOP_ApsSetData/64
  Ground/1 -> Data Type Conversion6/1
  Bus Selector3/1 -> R_HALOUT_TPMS_APS_CSOP_ApsSetData/1  "<VOUTP_PowerSta_enum>"
  Bus Selector3/81 -> Terminator13/1  "<VOUTP_VehSpeed_kph>"
  Bus Selector3/82 -> Terminator14/1  "<VOUTP_VehSpeed_kph>"
  Ground_12/1 -> Data Type Conversion119/1
  Bus Selector3/17 -> Data Type Conversion11/1  "<VOUTP_RFPulseCountV_flg>"
  Bus Selector3/18 -> Data Type Conversion12/1  "<VOUTP_LRPulseCountV_flg>"
  Bus Selector3/12 -> R_HALOUT_TPMS_APS_CSOP_ApsSetData/12  "<VOUTP_LFWhlRotDir_enum>"
  Bus Selector3/79 -> Terminator11/1  "<VOUTP_VehSpeed_kph>"
  Data Type Conversion117/1 -> R_HALOUT_TPMS_APS_CSOP_ApsSetData/83
  Bus Selector3/57 -> Data Type Conversion36/1  "<VOUTP_AVMErrSTA_flg>"
  Bus Selector3/40 -> Data Type Conversion25/1  "<VOUTP_LatAccelV_flg>"
  Bus Selector3/39 -> Data Type Conversion24/1  "<VOUTP_YawRateV_flg>"
  Bus Selector3/24 -> Terminator8/1  "<VOUTP_VehSpeed_kph>"
  Data Type Conversion35/1 -> R_HALOUT_TPMS_APS_CSOP_ApsSetData/53
  Bus Selector3/9 -> Data Type Conversion8/1  "<VOUTP_RFRawWhlSpeedV_flg>"
  Bus Selector3/83 -> Data Type Conversion117/1  "<VOUTP_IVIUserTakeOverAPSSta_flg>"
  Bus Selector3/55 -> R_HALOUT_TPMS_APS_CSOP_ApsSetData/55  "<VOUTP_AVMparkingexcute_enum>"
  Data Type Conversion10/1 -> R_HALOUT_TPMS_APS_CSOP_ApsSetData/16
  Bus Selector3/75 -> Terminator6/1  "<VOUTP_FSOffSwTimeOut_flg>"
  Bus Selector3/20 -> Data Type Conversion20/1  "<VOUTP_LFPulseCount_enum>"
  Bus Selector3/74 -> Terminator/1  "<VOUTP_FSOffSw_enum>"
  Bus Selector3/78 -> Terminator12/1  "<VOUTP_VehSpeed_kph>"
  Ground7/1 -> Data Type Conversion105/1
  Data Type Conversion32/1 -> R_HALOUT_TPMS_APS_CSOP_ApsSetData/48
  Data Type Conversion24/1 -> R_HALOUT_TPMS_APS_CSOP_ApsSetData/39
  Bus Selector3/47 -> Data Type Conversion31/1  "<VOUTP_EPBExtReleaseAvail_flg>"
  Data Type Conversion20/1 -> R_HALOUT_TPMS_APS_CSOP_ApsSetData/20
  Bus Selector3/19 -> Data Type Conversion13/1  "<VOUTP_RRPulseCountV_flg>"
  Data Type Conversion101/1 -> R_HALOUT_TPMS_APS_CSOP_ApsSetData/65
  Data Type Conversion103/1 -> R_HALOUT_TPMS_APS_CSOP_ApsSetData/63
  Data Type Conversion27/1 -> R_HALOUT_TPMS_APS_CSOP_ApsSetData/42
  Bus Selector3/6 -> R_HALOUT_TPMS_APS_CSOP_ApsSetData/6  "<VOUTP_LRRawWhlSpeed_kph>"
  Data Type Conversion104/1 -> R_HALOUT_TPMS_APS_CSOP_ApsSetData/62
  Bus Selector3/62 -> Data Type Conversion104/1  "<VOUTP_ABSActive_flg>"
  Bus Selector3/4 -> R_HALOUT_TPMS_APS_CSOP_ApsSetData/4  "<VOUTP_LFRawWhlSpeed_kph>"
  Bus Selector3/61 -> Terminator7/1  "<VOUTP_VehSpeedTimeOut_flg>"
  Bus Selector3/49 -> R_HALOUT_TPMS_APS_CSOP_ApsSetData/49  "<VOUTP_EPBErrSta_enum>"
  Data Type Conversion23/1 -> R_HALOUT_TPMS_APS_CSOP_ApsSetData/33
  Bus Selector3/54 -> R_HALOUT_TPMS_APS_CSOP_ApsSetData/54  "<VOUTP_AVMparkingcancel_enum>"
  Bus Selector3/59 -> R_HALOUT_TPMS_APS_CSOP_ApsSetData/59  "<VOUTP_CAASSw_enum>"
  Data Type Conversion13/1 -> R_HALOUT_TPMS_APS_CSOP_ApsSetData/19
  Bus Selector3/2 -> R_HALOUT_TPMS_APS_CSOP_ApsSetData/2  "<VOUTP_BrkPedalPos_pct>"
  Data Type Conversion28/1 -> R_HALOUT_TPMS_APS_CSOP_ApsSetData/43
  Data Type Conversion120/1 -> R_HALOUT_TPMS_APS_CSOP_ApsSetData/78
  Data Type Conversion15/1 -> R_HALOUT_TPMS_APS_CSOP_ApsSetData/22
  Bus Selector3/66 -> Data Type Conversion100/1  "<VOUTP_PsDoorSW_flg>"
  Bus Selector3/60 -> R_HALOUT_TPMS_APS_CSOP_ApsSetData/60  "<VOUTP_IVIScreen_enum>"
  Bus Selector3/64 -> Data Type Conversion102/1  "<VOUTP_DriverSeatBeltCmd_flg>"
  Bus Selector3/44 -> Data Type Conversion29/1  "<VOUTP_BrkSwV_flg>"
  Bus Selector3/13 -> R_HALOUT_TPMS_APS_CSOP_ApsSetData/13  "<VOUTP_RFWhlRotDir_enum>"
  Bus Selector3/22 -> Data Type Conversion15/1  "<VOUTP_LRPulseCount_enum>"
  Bus Selector3/28 -> R_HALOUT_TPMS_APS_CSOP_ApsSetData/28  "<VOUTP_EPSAOIControl_enum>"
  Bus Selector3/26 -> R_HALOUT_TPMS_APS_CSOP_ApsSetData/26  "<VOUTP_ShifterHandleCmd_enum>"
  Bus Selector3/69 -> R_HALOUT_TPMS_APS_CSOP_ApsSetData/69  "<VOUTP_RFPressIndi_enum>"
  Bus Selector3/3 -> R_HALOUT_TPMS_APS_CSOP_ApsSetData/3  "<VOUTP_ActAPSPosn_pct>"
  Ground_13/1 -> Data Type Conversion120/1
  Data Type Conversion11/1 -> R_HALOUT_TPMS_APS_CSOP_ApsSetData/17
  Data Type Conversion119/1 -> R_HALOUT_TPMS_APS_CSOP_ApsSetData/77
  Data Type Conversion16/1 -> R_HALOUT_TPMS_APS_CSOP_ApsSetData/23
  Data Type Conversion14/1 -> R_HALOUT_TPMS_APS_CSOP_ApsSetData/21
  Bus Selector3/33 -> Data Type Conversion23/1  "<VOUTP_SASV_flg>"
  Data Type Conversion33/1 -> R_HALOUT_TPMS_APS_CSOP_ApsSetData/51
  Data Type Conversion34/1 -> R_HALOUT_TPMS_APS_CSOP_ApsSetData/52
  [BOUTP_outputs] -> Bus Selector3/1
  Bus Selector3/37 -> R_HALOUT_TPMS_APS_CSOP_ApsSetData/37  "<VOUTP_LongAccel_Gps>"
  Bus Selector3/41 -> Data Type Conversion26/1  "<VOUTP_LongAccelV_flg>"
  Bus Selector3/65 -> Data Type Conversion101/1  "<VOUTP_DrDoorSW_flg>"
  Data Type Conversion25/1 -> R_HALOUT_TPMS_APS_CSOP_ApsSetData/40
  Bus Selector3/30 -> R_HALOUT_TPMS_APS_CSOP_ApsSetData/30  "<VOUTP_SASSpeed_degps>"
  Bus Selector3/53 -> Data Type Conversion35/1  "<VOUTP_TailgateSW_flg>"
  Bus Selector3/42 -> Data Type Conversion27/1  "<VOUTP_MCPressureV_bar>"
  Data Type Conversion21/1 -> R_HALOUT_TPMS_APS_CSOP_ApsSetData/31
  Bus Selector3/5 -> R_HALOUT_TPMS_APS_CSOP_ApsSetData/5  "<VOUTP_RFRawWhlSpeed_kph>"
  Ground_17/1 -> Data Type Conversion124/1
  Bus Selector3/48 -> Data Type Conversion32/1  "<VOUTP_EPBExtApplyAvail_flg>"
  Data Type Conversion19/1 -> R_HALOUT_TPMS_APS_CSOP_ApsSetData/11
  Bus Selector3/45 -> Data Type Conversion30/1  "<VOUTP_ESCStandstill_flg>"
  Data Type Conversion17/1 -> R_HALOUT_TPMS_APS_CSOP_ApsSetData/24
  Data Type Conversion98/1 -> R_HALOUT_TPMS_APS_CSOP_ApsSetData/68
  Bus Selector3/58 -> Data Type Conversion37/1  "<VOUTP_IVIStatus_flg>"
  Bus Selector3/63 -> Data Type Conversion103/1  "<VOUTP_TCSActive_flg>"
  Bus Selector3/11 -> Data Type Conversion19/1  "<VOUTP_RRRawWhlSpeedV_flg>"
  Bus Selector3/16 -> Data Type Conversion10/1  "<VOUTP_LFPulseCountV_flg>"
  Data Type Conversion7/1 -> R_HALOUT_TPMS_APS_CSOP_ApsSetData/8
  Bus Selector3/51 -> Data Type Conversion33/1  "<VOUTP_AllDoorSW_flg>"
  Bus Selector3/43 -> Data Type Conversion28/1  "<VOUTP_BrkSwSta_flg>"
  Data Type Conversion26/1 -> R_HALOUT_TPMS_APS_CSOP_ApsSetData/41
  Bus Selector3/70 -> R_HALOUT_TPMS_APS_CSOP_ApsSetData/70  "<VOUTP_LFPressIndi_enum>"
  Bus Selector3/29 -> R_HALOUT_TPMS_APS_CSOP_ApsSetData/29  "<VOUTP_SASAngle_Deg>"
  Ground8/1 -> Data Type Conversion17/1
  Ground_16/1 -> Data Type Conversion122/1
  Data Type Conversion30/1 -> R_HALOUT_TPMS_APS_CSOP_ApsSetData/45
  Data Type Conversion37/1 -> R_HALOUT_TPMS_APS_CSOP_ApsSetData/58
  Data Type Conversion122/1 -> R_HALOUT_TPMS_APS_CSOP_ApsSetData/81
  Bus Selector3/72 -> R_HALOUT_TPMS_APS_CSOP_ApsSetData/72  "<VOUTP_LRPressIndi_enum>"
  Bus Selector3/31 -> Data Type Conversion21/1  "<VOUTP_SASSpeedValid_flg>"
  Data Type Conversion9/1 -> R_HALOUT_TPMS_APS_CSOP_ApsSetData/10
  Bus Selector3/25 -> Data Type Conversion18/1  "<VOUTP_APSCtrlAvail_flg>"
  Bus Selector3/21 -> Data Type Conversion14/1  "<VOUTP_RFPulseCount_enum>"
  Bus Selector3/76 -> Terminator15/1  "<VOUTP_VehSpeed_kph>"
  Ground_11/1 -> Data Type Conversion118/1
  Data Type Conversion29/1 -> R_HALOUT_TPMS_APS_CSOP_ApsSetData/44
  Bus Selector3/56 -> R_HALOUT_TPMS_APS_CSOP_ApsSetData/56  "<VOUTP_AVMParkingmode_enum>"
  Bus Selector3/80 -> R_HALOUT_TPMS_APS_CSOP_ApsSetData/80  "<VOUTP_DrSeatSta_enum>"
  Ground_14/1 -> Data Type Conversion121/1
  Data Type Conversion124/1 -> R_HALOUT_TPMS_APS_CSOP_ApsSetData/82
  Data Type Conversion12/1 -> R_HALOUT_TPMS_APS_CSOP_ApsSetData/18
  Bus Selector3/23 -> Data Type Conversion16/1  "<VOUTP_RRPulseCount_enum>"
  Bus Selector3/67 -> Data Type Conversion99/1  "<VOUTP_RLDoorSW_flg>"
  Bus Selector3/35 -> R_HALOUT_TPMS_APS_CSOP_ApsSetData/35  "<VOUTP_YawRate_degps>"
  Bus Selector3/14 -> R_HALOUT_TPMS_APS_CSOP_ApsSetData/14  "<VOUTP_LRWhlRotDir_enum>"
  Bus Selector3/77 -> Terminator10/1  "<VOUTP_VehSpeed_kph>"
  Bus Selector3/10 -> Data Type Conversion9/1  "<VOUTP_LRRawWhlSpeedV_flg>"
  Bus Selector3/32 -> Data Type Conversion22/1  "<VOUTP_SASCAL_flg>"
  Data Type Conversion31/1 -> R_HALOUT_TPMS_APS_CSOP_ApsSetData/47
  Bus Selector3/34 -> R_HALOUT_TPMS_APS_CSOP_ApsSetData/34  "<VOUTP_GRADE_Deg>"
  Data Type Conversion118/1 -> R_HALOUT_TPMS_APS_CSOP_ApsSetData/76
  Bus Selector3/52 -> Data Type Conversion34/1  "<VOUTP_HoodSW_flg>"
  Bus Selector3/46 -> R_HALOUT_TPMS_APS_CSOP_ApsSetData/46  "<VOUTP_ESCAPSSta_enum>"
  Data Type Conversion36/1 -> R_HALOUT_TPMS_APS_CSOP_ApsSetData/57
  Ground6/1 -> Data Type Conversion96/1
  Data Type Conversion18/1 -> R_HALOUT_TPMS_APS_CSOP_ApsSetData/25
  Data Type Conversion6/1 -> R_HALOUT_TPMS_APS_CSOP_ApsSetData/74
  Data Type Conversion22/1 -> R_HALOUT_TPMS_APS_CSOP_ApsSetData/32
  Bus Selector3/68 -> Data Type Conversion98/1  "<VOUTP_RRDoorSW_flg>"
  Data Type Conversion105/1 -> R_HALOUT_TPMS_APS_CSOP_ApsSetData/61
  Bus Selector3/50 -> R_HALOUT_TPMS_APS_CSOP_ApsSetData/50  "<VOUTP_EPBSta_enum>"
  Bus Selector3/73 -> R_HALOUT_TPMS_APS_CSOP_ApsSetData/73  "<VOUTP_sigAmbAirT_C>"
  Bus Selector3/27 -> R_HALOUT_TPMS_APS_CSOP_ApsSetData/27  "<VOUTP_DriIntend_enum>"
  Data Type Conversion8/1 -> R_HALOUT_TPMS_APS_CSOP_ApsSetData/9
  Bus Selector3/15 -> R_HALOUT_TPMS_APS_CSOP_ApsSetData/15  "<VOUTP_RRWhlRotDir_enum>"
  Data Type Conversion96/1 -> R_HALOUT_TPMS_APS_CSOP_ApsSetData/75
  Bus Selector3/36 -> R_HALOUT_TPMS_APS_CSOP_ApsSetData/36  "<VOUTP_LatAccel_Gps>"
  Bus Selector3/38 -> R_HALOUT_TPMS_APS_CSOP_ApsSetData/38  "<VOUTP_MCPressure_bar>"
  Bus Selector3/7 -> R_HALOUT_TPMS_APS_CSOP_ApsSetData/7  "<VOUTP_RRRawWhlSpeed_kph>"
  Data Type Conversion100/1 -> R_HALOUT_TPMS_APS_CSOP_ApsSetData/66
  Bus Selector3/71 -> R_HALOUT_TPMS_APS_CSOP_ApsSetData/71  "<VOUTP_RRPressIndi_enum>"
  Data Type Conversion121/1 -> R_HALOUT_TPMS_APS_CSOP_ApsSetData/79
  Data Type Conversion61/1 -> R_HALOUT_TPMS_APS_CSOP_ApsSetTimeout/27
  Data Type Conversion88/1 -> R_HALOUT_TPMS_APS_CSOP_ApsSetTimeout/52
  Ground_19/1 -> Data Type Conversion113/1
  Data Type Conversion46/1 -> R_HALOUT_TPMS_APS_CSOP_ApsSetTimeout/12
  Data Type Conversion93/1 -> R_HALOUT_TPMS_APS_CSOP_ApsSetTimeout/60
  Data Type Conversion48/1 -> R_HALOUT_TPMS_APS_CSOP_ApsSetTimeout/15
  Ground3/1 -> Data Type Conversion94/1
  Data Type Conversion70/1 -> R_HALOUT_TPMS_APS_CSOP_ApsSetTimeout/37
  Data Type Conversion110/1 -> R_HALOUT_TPMS_APS_CSOP_ApsSetTimeout/66
  Data Type Conversion85/1 -> R_HALOUT_TPMS_APS_CSOP_ApsSetTimeout/55
  Data Type Conversion97/1 -> R_HALOUT_TPMS_APS_CSOP_ApsSetTimeout/50
  Ground1/1 -> Data Type Conversion92/1
  Data Type Conversion58/1 -> R_HALOUT_TPMS_APS_CSOP_ApsSetTimeout/24
  Data Type Conversion75/1 -> R_HALOUT_TPMS_APS_CSOP_ApsSetTimeout/38
  Data Type Conversion82/1 -> R_HALOUT_TPMS_APS_CSOP_ApsSetTimeout/54
  Data Type Conversion39/1 -> R_HALOUT_TPMS_APS_CSOP_ApsSetTimeout/5
  Data Type Conversion109/1 -> R_HALOUT_TPMS_APS_CSOP_ApsSetTimeout/62
  Data Type Conversion106/1 -> R_HALOUT_TPMS_APS_CSOP_ApsSetTimeout/57
  Data Type Conversion92/1 -> R_HALOUT_TPMS_APS_CSOP_ApsSetTimeout/61
  Ground_21/1 -> Data Type Conversion111/1
  Data Type Conversion51/1 -> R_HALOUT_TPMS_APS_CSOP_ApsSetTimeout/3
  Ground2/1 -> Data Type Conversion93/1
  Ground_23/1 -> Data Type Conversion116/1
  Data Type Conversion56/1 -> R_HALOUT_TPMS_APS_CSOP_ApsSetTimeout/13
  Data Type Conversion50/1 -> R_HALOUT_TPMS_APS_CSOP_ApsSetTimeout/17
  Data Type Conversion38/1 -> R_HALOUT_TPMS_APS_CSOP_ApsSetTimeout/4
  Data Type Conversion78/1 -> R_HALOUT_TPMS_APS_CSOP_ApsSetTimeout/44
  Data Type Conversion52/1 -> R_HALOUT_TPMS_APS_CSOP_ApsSetTimeout/19
  Data Type Conversion69/1 -> R_HALOUT_TPMS_APS_CSOP_ApsSetTimeout/36
  Data Type Conversion43/1 -> R_HALOUT_TPMS_APS_CSOP_ApsSetTimeout/10
  Data Type Conversion89/1 -> R_HALOUT_TPMS_APS_CSOP_ApsSetTimeout/53
  Data Type Conversion49/1 -> R_HALOUT_TPMS_APS_CSOP_ApsSetTimeout/16
  Data Type Conversion74/1 -> R_HALOUT_TPMS_APS_CSOP_ApsSetTimeout/41
  Data Type Conversion64/1 -> R_HALOUT_TPMS_APS_CSOP_ApsSetTimeout/31
  Data Type Conversion83/1 -> R_HALOUT_TPMS_APS_CSOP_ApsSetTimeout/47
  Data Type Conversion72/1 -> R_HALOUT_TPMS_APS_CSOP_ApsSetTimeout/39
  Data Type Conversion95/1 -> R_HALOUT_TPMS_APS_CSOP_ApsSetTimeout/58
  Data Type Conversion59/1 -> R_HALOUT_TPMS_APS_CSOP_ApsSetTimeout/25
  Data Type Conversion45/1 -> R_HALOUT_TPMS_APS_CSOP_ApsSetTimeout/8
  Data Type Conversion67/1 -> R_HALOUT_TPMS_APS_CSOP_ApsSetTimeout/34
  Data Type Conversion76/1 -> R_HALOUT_TPMS_APS_CSOP_ApsSetTimeout/33
  Data Type Conversion79/1 -> R_HALOUT_TPMS_APS_CSOP_ApsSetTimeout/45
  Data Type Conversion53/1 -> R_HALOUT_TPMS_APS_CSOP_ApsSetTimeout/20
  Data Type Conversion60/1 -> R_HALOUT_TPMS_APS_CSOP_ApsSetTimeout/26
  Data Type Conversion94/1 -> R_HALOUT_TPMS_APS_CSOP_ApsSetTimeout/59
  Data Type Conversion90/1 -> R_HALOUT_TPMS_APS_CSOP_ApsSetTimeout/56
  Data Type Conversion65/1 -> R_HALOUT_TPMS_APS_CSOP_ApsSetTimeout/28
  Data Type Conversion116/1 -> R_HALOUT_TPMS_APS_CSOP_ApsSetTimeout/67
  Data Type Conversion113/1 -> R_HALOUT_TPMS_APS_CSOP_ApsSetTimeout/63
  Ground_20/1 -> Data Type Conversion112/1
  Ground_26/1 -> Data Type Conversion114/1
  Data Type Conversion44/1 -> R_HALOUT_TPMS_APS_CSOP_ApsSetTimeout/11
  Data Type Conversion42/1 -> R_HALOUT_TPMS_APS_CSOP_ApsSetTimeout/9
  Ground5/1 -> Data Type Conversion106/1
  Data Type Conversion73/1 -> R_HALOUT_TPMS_APS_CSOP_ApsSetTimeout/40
  Data Type Conversion114/1 -> R_HALOUT_TPMS_APS_CSOP_ApsSetTimeout/69
  Ground_24/1 -> Data Type Conversion115/1
  Data Type Conversion111/1 -> R_HALOUT_TPMS_APS_CSOP_ApsSetTimeout/65
  Data Type Conversion80/1 -> R_HALOUT_TPMS_APS_CSOP_ApsSetTimeout/46
  Data Type Conversion62/1 -> R_HALOUT_TPMS_APS_CSOP_ApsSetTimeout/29
  Data Type Conversion57/1 -> R_HALOUT_TPMS_APS_CSOP_ApsSetTimeout/22
  Data Type Conversion91/1 -> R_HALOUT_TPMS_APS_CSOP_ApsSetTimeout/43
  Data Type Conversion66/1 -> R_HALOUT_TPMS_APS_CSOP_ApsSetTimeout/32
  Data Type Conversion81/1 -> R_HALOUT_TPMS_APS_CSOP_ApsSetTimeout/1
  Data Type Conversion68/1 -> R_HALOUT_TPMS_APS_CSOP_ApsSetTimeout/35
  Data Type Conversion47/1 -> R_HALOUT_TPMS_APS_CSOP_ApsSetTimeout/14
  Data Type Conversion40/1 -> R_HALOUT_TPMS_APS_CSOP_ApsSetTimeout/6
  Data Type Conversion71/1 -> R_HALOUT_TPMS_APS_CSOP_ApsSetTimeout/23
  Data Type Conversion84/1 -> R_HALOUT_TPMS_APS_CSOP_ApsSetTimeout/48
  Data Type Conversion63/1 -> R_HALOUT_TPMS_APS_CSOP_ApsSetTimeout/30
  Data Type Conversion54/1 -> R_HALOUT_TPMS_APS_CSOP_ApsSetTimeout/21
  Data Type Conversion112/1 -> R_HALOUT_TPMS_APS_CSOP_ApsSetTimeout/64
  Ground4/1 -> Data Type Conversion95/1
  Data Type Conversion77/1 -> R_HALOUT_TPMS_APS_CSOP_ApsSetTimeout/42
  Data Type Conversion87/1 -> R_HALOUT_TPMS_APS_CSOP_ApsSetTimeout/51
  Data Type Conversion123/1 -> R_HALOUT_TPMS_APS_CSOP_ApsSetTimeout/2
  Ground_22/1 -> Data Type Conversion110/1
  Data Type Conversion41/1 -> R_HALOUT_TPMS_APS_CSOP_ApsSetTimeout/7
  Data Type Conversion86/1 -> R_HALOUT_TPMS_APS_CSOP_ApsSetTimeout/49
  Data Type Conversion55/1 -> R_HALOUT_TPMS_APS_CSOP_ApsSetTimeout/18
  Data Type Conversion115/1 -> R_HALOUT_TPMS_APS_CSOP_ApsSetTimeout/68
  R_BOUTP2_outputs_BOUTP2_outputs_read/1 -> [BOUTP_outputs]
  Data Type Conversion/1 -> IRV_f32_ApsOutVehSpdSig_write/1
  Bus Selector/4 -> Data Type Conversion3/1  "<VOUTP_VehSpeedTimeOut_flg>"
  Bus Selector/5 -> Data Type Conversion4/1  "<VOUTP_FSOffSwTimeOut_flg>"
  Data Type Conversion5/1 -> IRV_u8_ApsOutSetVehSpdTOCmd_write/1
  Bus Selector/6 -> Data Type Conversion5/1  "<VOUTP_ChrgPlugSta_enum>"
  [BOUTP_outputs] -> Bus Selector/1
  Data Type Conversion2/1 -> IRV_u8_ApsOutSendChrgPlugSta_write/1
  Data Type Conversion1/1 -> IRV_u8_ApsOutGearPosnSig_write/1
  Data Type Conversion3/1 -> IRV_u8_ApsOutSetFrSensorOnCmd_write/1
  Bus Selector/3 -> Data Type Conversion2/1  "<VOUTP_FSOffSw_enum>"
  Bus Selector/2 -> Data Type Conversion1/1  "<VOUTP_ShiftGearPosn_enum>"
  Bus Selector/1 -> Data Type Conversion/1  "<VOUTP_VehSpeed_kph>"
  Data Type Conversion4/1 -> IRV_u8_ApsOutSetFrSensorSwTOCmd_write/1
  Ground_1/1 -> Data Type Conversion109/1
  Ground_2/1 -> Data Type Conversion86/1
  Ground_6/1 -> Data Type Conversion89/1
  Ground12/1 -> Data Type Conversion79/1
  Ground_8/1 -> Data Type Conversion85/1
  Ground13/1 -> Data Type Conversion78/1
  Ground_9/1 -> Data Type Conversion90/1
  Ground_4/1 -> Data Type Conversion87/1
  Ground_7/1 -> Data Type Conversion82/1
  Ground10/1 -> Data Type Conversion83/1
  Ground_5/1 -> Data Type Conversion88/1
  Ground9/1 -> Data Type Conversion84/1
  Ground11/1 -> Data Type Conversion80/1
  Ground_3/1 -> Data Type Conversion97/1
  Ground_32/1 -> Data Type Conversion58/1
  Ground16/1 -> Data Type Conversion53/1
  Ground23/1 -> Data Type Conversion57/1
  Ground_34/1 -> Data Type Conversion60/1
  Ground15/1 -> Data Type Conversion54/1
  Ground_36/1 -> Data Type Conversion65/1
  Ground_33/1 -> Data Type Conversion59/1
  Ground_38/1 -> Data Type Conversion63/1
  Ground18/1 -> Data Type Conversion55/1
  Ground_37/1 -> Data Type Conversion62/1
  Ground17/1 -> Data Type Conversion52/1
  Ground_35/1 -> Data Type Conversion61/1
  Ground_18/1 -> Data Type Conversion71/1
  Ground_10/1 -> Data Type Conversion69/1
  Ground_28/1 -> Data Type Conversion73/1
  Ground21/1 -> Data Type Conversion66/1
  Ground_30/1 -> Data Type Conversion77/1
  Ground22/1 -> Data Type Conversion64/1
  Ground_31/1 -> Data Type Conversion91/1
  Ground_25/1 -> Data Type Conversion75/1
  Ground_29/1 -> Data Type Conversion74/1
  Ground19/1 -> Data Type Conversion67/1
  Ground_27/1 -> Data Type Conversion72/1
  Ground14/1 -> Data Type Conversion68/1
  Ground20/1 -> Data Type Conversion76/1
  Ground_15/1 -> Data Type Conversion70/1
  Ground28/1 -> Data Type Conversion50/1
  Ground_39/1 -> Data Type Conversion42/1
  Ground_43/1 -> Data Type Conversion56/1
  Ground26/1 -> Data Type Conversion39/1
  Ground_45/1 -> Data Type Conversion48/1
  Ground27/1 -> Data Type Conversion38/1
  Ground_46/1 -> Data Type Conversion49/1
  Ground_41/1 -> Data Type Conversion44/1
  Ground_44/1 -> Data Type Conversion47/1
  Ground24/1 -> Data Type Conversion41/1
  Ground_42/1 -> Data Type Conversion46/1
  Ground29/1 -> Data Type Conversion45/1
  Ground25/1 -> Data Type Conversion40/1
  Ground_40/1 -> Data Type Conversion43/1
  Ground31/1 -> Data Type Conversion123/1
  Ground30/1 -> Data Type Conversion51/1
  Ground32/1 -> Data Type Conversion81/1

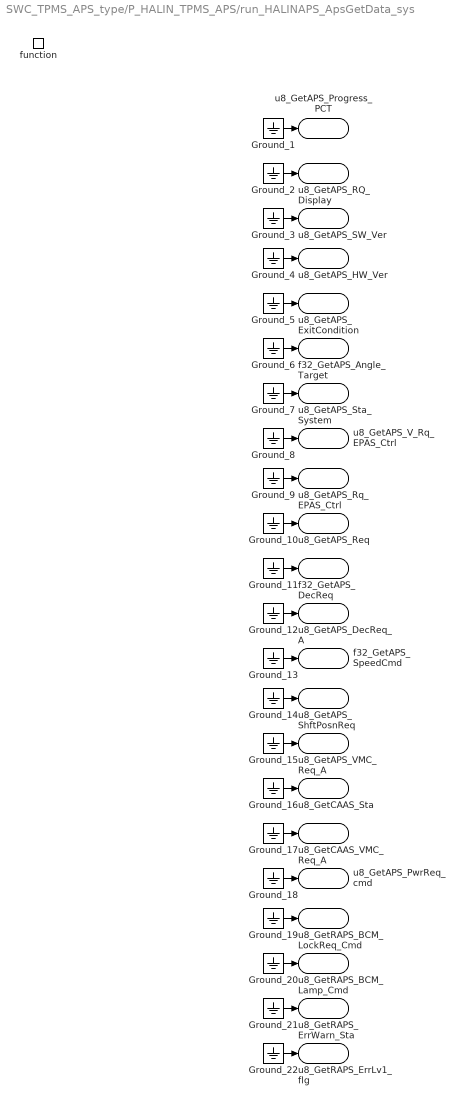
== system SWC_TPMS_APS_type/P_HALIN_TPMS_APS/run_HALINAPS_ApsGetData_sys ==
  function : TriggerPort  TriggerType=function-call  IsSimulinkFunction=on  FunctionName=run_HALINAPS_ApsGetData  VariantControl=(inherit)
  Ground_{1..22} (22 alike) : Ground
  u8_GetAPS_Progress_PCT : ArgOut  OutDataTypeStr=uint8  ArgumentName=u8_GetAPS_Progress_PCT
  u8_GetAPS_RQ_Display : ArgOut  Port=2  OutDataTypeStr=uint8  ArgumentName=u8_GetAPS_RQ_Display
  u8_GetAPS_SW_Ver : ArgOut  Port=3  OutDataTypeStr=uint8  ArgumentName=u8_GetAPS_SW_Ver
  u8_GetAPS_HW_Ver : ArgOut  Port=4  OutDataTypeStr=uint8  ArgumentName=u8_GetAPS_HW_Ver
  u8_GetAPS_ExitCondition : ArgOut  Port=5  OutDataTypeStr=uint8  ArgumentName=u8_GetAPS_ExitCondition
  f32_GetAPS_Angle_Target : ArgOut  Port=6  OutDataTypeStr=single  ArgumentName=f32_GetAPS_Angle_Target
  u8_GetAPS_Sta_System : ArgOut  Port=7  OutDataTypeStr=uint8  ArgumentName=u8_GetAPS_Sta_System
  u8_GetAPS_V_Rq_EPAS_Ctrl : ArgOut  Port=8  OutDataTypeStr=uint8  ArgumentName=u8_GetAPS_V_Rq_EPAS_Ctrl
  u8_GetAPS_Rq_EPAS_Ctrl : ArgOut  Port=9  OutDataTypeStr=uint8  ArgumentName=u8_GetAPS_Rq_EPAS_Ctrl
  u8_GetAPS_Req : ArgOut  Port=10  OutDataTypeStr=uint8  ArgumentName=u8_GetAPS_Req
  f32_GetAPS_DecReq : ArgOut  Port=11  OutDataTypeStr=single  ArgumentName=f32_GetAPS_DecReq
  u8_GetAPS_DecReq_A : ArgOut  Port=12  OutDataTypeStr=uint8  ArgumentName=u8_GetAPS_DecReq_A
  f32_GetAPS_SpeedCmd : ArgOut  Port=13  OutDataTypeStr=single  ArgumentName=f32_GetAPS_SpeedCmd
  u8_GetAPS_ShftPosnReq : ArgOut  Port=14  OutDataTypeStr=uint8  ArgumentName=u8_GetAPS_ShftPosnReq
  u8_GetAPS_VMC_Req_A : ArgOut  Port=15  OutDataTypeStr=uint8  ArgumentName=u8_GetAPS_VMC_Req_A
  u8_GetCAAS_Sta : ArgOut  Port=16  OutDataTypeStr=uint8  ArgumentName=u8_GetCAAS_Sta
  u8_GetCAAS_VMC_Req_A : ArgOut  Port=17  OutDataTypeStr=uint8  ArgumentName=u8_GetCAAS_VMC_Req_A
  u8_GetAPS_PwrReq_cmd : ArgOut  Port=18  OutDataTypeStr=uint8  ArgumentName=u8_GetAPS_PwrReq_cmd
  u8_GetRAPS_BCM_LockReq_Cmd : ArgOut  Port=19  OutDataTypeStr=uint8  ArgumentName=u8_GetRAPS_BCM_LockReq_Cmd
  u8_GetRAPS_BCM_Lamp_Cmd : ArgOut  Port=20  OutDataTypeStr=uint8  ArgumentName=u8_GetRAPS_BCM_Lamp_Cmd
  u8_GetRAPS_ErrWarn_Sta : ArgOut  Port=21  OutDataTypeStr=uint8  ArgumentName=u8_GetRAPS_ErrWarn_Sta
  u8_GetRAPS_ErrLv1_flg : ArgOut  Port=22  OutDataTypeStr=uint8  ArgumentName=u8_GetRAPS_ErrLv1_flg
  wires:
  Ground_1/1 -> u8_GetAPS_Progress_PCT/1
  Ground_2/1 -> u8_GetAPS_RQ_Display/1
  Ground_3/1 -> u8_GetAPS_SW_Ver/1
  Ground_4/1 -> u8_GetAPS_HW_Ver/1
  Ground_5/1 -> u8_GetAPS_ExitCondition/1
  Ground_6/1 -> f32_GetAPS_Angle_Target/1
  Ground_7/1 -> u8_GetAPS_Sta_System/1
  Ground_8/1 -> u8_GetAPS_V_Rq_EPAS_Ctrl/1
  Ground_9/1 -> u8_GetAPS_Rq_EPAS_Ctrl/1
  Ground_10/1 -> u8_GetAPS_Req/1
  Ground_11/1 -> f32_GetAPS_DecReq/1
  Ground_12/1 -> u8_GetAPS_DecReq_A/1
  Ground_13/1 -> f32_GetAPS_SpeedCmd/1
  Ground_14/1 -> u8_GetAPS_ShftPosnReq/1
  Ground_15/1 -> u8_GetAPS_VMC_Req_A/1
  Ground_16/1 -> u8_GetCAAS_Sta/1
  Ground_17/1 -> u8_GetCAAS_VMC_Req_A/1
  Ground_18/1 -> u8_GetAPS_PwrReq_cmd/1
  Ground_19/1 -> u8_GetRAPS_BCM_LockReq_Cmd/1
  Ground_20/1 -> u8_GetRAPS_BCM_Lamp_Cmd/1
  Ground_21/1 -> u8_GetRAPS_ErrWarn_Sta/1
  Ground_22/1 -> u8_GetRAPS_ErrLv1_flg/1

== system SWC_TPMS_APS_type/P_HALIN_TPMS_APS/run_HALINAPS_ApsGetDistLevel_sys ==
  function : TriggerPort  TriggerType=function-call  IsSimulinkFunction=on  FunctionName=run_HALINAPS_ApsGetDistLevel  VariantControl=(inherit)
  Ground_1 : Ground
  u8Array8_ApsInLevel : ArgOut  OutDataTypeStr=uint8  PortDimensions=8  ArgumentName=u8Array8_ApsInLevel
  wires:
  Ground_1/1 -> u8Array8_ApsInLevel/1

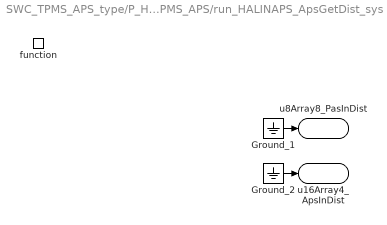
== system SWC_TPMS_APS_type/P_HALIN_TPMS_APS/run_HALINAPS_ApsGetDist_sys ==
  function : TriggerPort  TriggerType=function-call  IsSimulinkFunction=on  FunctionName=run_HALINAPS_ApsGetDist  VariantControl=(inherit)
  Ground_1 : Ground
  Ground_2 : Ground
  u8Array8_PasInDist : ArgOut  OutDataTypeStr=uint8  PortDimensions=8  ArgumentName=u8Array8_PasInDist
  u16Array4_ApsInDist : ArgOut  Port=2  OutDataTypeStr=uint16  PortDimensions=4  ArgumentName=u16Array4_ApsInDist
  wires:
  Ground_1/1 -> u8Array8_PasInDist/1
  Ground_2/1 -> u16Array4_ApsInDist/1

== system SWC_TPMS_APS_type/P_HALIN_TPMS_APS/run_HALINAPS_ApsGetUssSta_sys ==
  function : TriggerPort  TriggerType=function-call  IsSimulinkFunction=on  FunctionName=run_HALINAPS_ApsGetUssSta  VariantControl=(inherit)
  Ground_1 : Ground
  u8Array12_ApsInUssSta : ArgOut  OutDataTypeStr=uint8  PortDimensions=12  ArgumentName=u8Array12_ApsInUssSta
  wires:
  Ground_1/1 -> u8Array12_ApsInUssSta/1

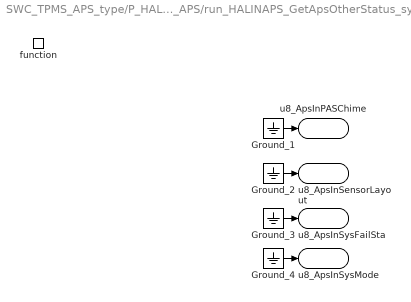
== system SWC_TPMS_APS_type/P_HALIN_TPMS_APS/run_HALINAPS_GetApsOtherStatus_sys ==
  function : TriggerPort  TriggerType=function-call  IsSimulinkFunction=on  FunctionName=run_HALINAPS_GetApsOtherStatus  VariantControl=(inherit)
  Ground_{1..4} (4 alike) : Ground
  u8_ApsInPASChime : ArgOut  OutDataTypeStr=uint8  ArgumentName=u8_ApsInPASChime
  u8_ApsInSensorLayout : ArgOut  Port=2  OutDataTypeStr=uint8  ArgumentName=u8_ApsInSensorLayout
  u8_ApsInSysFailSta : ArgOut  Port=3  OutDataTypeStr=uint8  ArgumentName=u8_ApsInSysFailSta
  u8_ApsInSysMode : ArgOut  Port=4  OutDataTypeStr=uint8  ArgumentName=u8_ApsInSysMode
  wires:
  Ground_1/1 -> u8_ApsInPASChime/1
  Ground_2/1 -> u8_ApsInSensorLayout/1
  Ground_3/1 -> u8_ApsInSysFailSta/1
  Ground_4/1 -> u8_ApsInSysMode/1

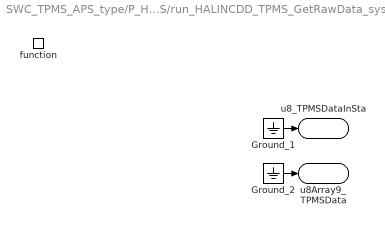
== system SWC_TPMS_APS_type/P_HALIN_TPMS_APS/run_HALINCDD_TPMS_GetRawData_sys ==
  function : TriggerPort  TriggerType=function-call  IsSimulinkFunction=on  FunctionName=run_HALINCDD_TPMS_GetRawData  VariantControl=(inherit)
  Ground_1 : Ground
  Ground_2 : Ground
  u8_TPMSDataInSta : ArgOut  OutDataTypeStr=uint8  ArgumentName=u8_TPMSDataInSta
  u8Array9_TPMSData : ArgOut  Port=2  OutDataTypeStr=uint8  PortDimensions=9  ArgumentName=u8Array9_TPMSData
  wires:
  Ground_1/1 -> u8_TPMSDataInSta/1
  Ground_2/1 -> u8Array9_TPMSData/1

== system SWC_TPMS_APS_type/P_HALIN_TPMS_APS/run_PAS_Handler_sys ==
  function : TriggerPort  TriggerType=function-call  IsSimulinkFunction=on  FunctionName=run_PAS_Handler  VariantControl=(inherit)

== system SWC_TPMS_APS_type/P_HALIN_TPMS_APS/run_TPMS_Handler_sys ==
  note: Added blocks
  function : TriggerPort  TriggerType=function-call  IsSimulinkFunction=on  FunctionName=run_TPMS_Handler  VariantControl=(inherit)
